simulink model "FFPID"  (R2024a)
settings: Solver=ode45  StartTime=0.0  StopTime=20  FixedStep=1e-2  RelTol=1e-4  AbsTol=1e-4
values from neighbouring files (symbols this model uses):
  constraint = 100    [single_ITAE.m]
undefined symbols (not defined in the file or in its folder): Kff, Kp, Td, Ti
libraries: cstblocks x2
settings Model: Creator=bhir  LastModifiedBy=Flo
settings SolverCC: AlgebraicLoopSolver=TrustRegion
settings DataIOCC: ReturnWorkspaceOutputs=off
settings DebuggingCC: UnconnectedInputMsg=warning  UnconnectedOutputMsg=warning  UnconnectedLineMsg=warning  ArithmeticOperatorsInVariantConditions=warning
settings SFSimCC: SimUseLocalCustomCode=off  CustomCodeUndefinedFunction=UseInterfaceOnly
settings RTWCC: RTWUseLocalCustomCode=off  GPUComputeCapability=3.5  DLArmComputeVersion=19.05
settings CodeAppCC: StateflowObjectComments=on

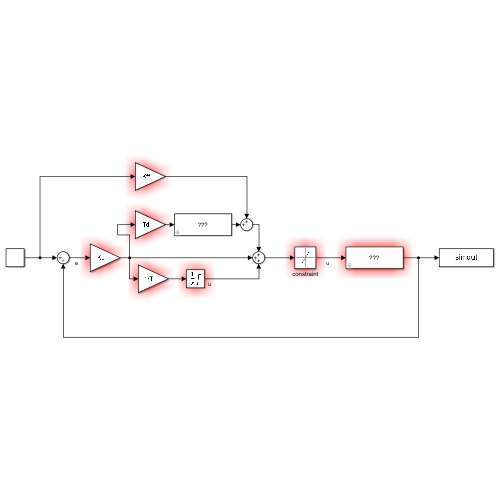
[thumbnail: Simulink's stored preview of the top-level diagram]
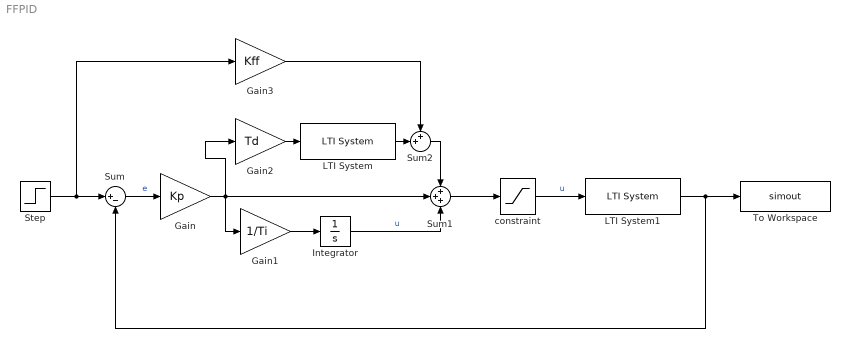
== system FFPID ==
  Gain : Gain  Gain=Kp
  Gain1 : Gain  Gain=1/Ti
  Gain2 : Gain  Gain=Td
  Gain3 : Gain  Gain=Kff
  Integrator : Integrator  LimitOutput=on  UpperSaturationLimit=constraint  LowerSaturationLimit=-constraint
  LTI System : cstblocks/LTI System  sys=filter  IC=[]  PadeOrder=0
  LTI System1 : cstblocks/LTI System  sys=plant  IC=[]  PadeOrder=0
  Step : Step  Time=0  SampleTime=0
  Sum : Sum  Inputs=|+-
  Sum1 : Sum  Inputs=+++
  Sum2 : Sum  Inputs=++|
  To Workspace : ToWorkspace  VariableName=simout  SaveFormat=Structure With Time  SampleTime=-1
  constraint : Saturate  UpperLimit=constraint  LowerLimit=-constraint
  wires:
  Step/1 -> Gain3/1, Sum/1
  Sum/1 -> Gain/1  "e"
  Gain/1 -> Gain1/1, Gain2/1, Sum1/2
  Gain2/1 -> LTI System/1
  Sum1/1 -> constraint/1
  constraint/1 -> LTI System1/1  "u"
  LTI System1/1 -> To Workspace/1, Sum/2
  Gain1/1 -> Integrator/1
  Integrator/1 -> Sum1/3  "u"
  Gain3/1 -> Sum2/1
  LTI System/1 -> Sum2/2
  Sum2/1 -> Sum1/1
